simulink model "Test"  (R2022b)
settings: Solver=VariableStepAuto  StartTime=0.0  StopTime=500  MaxStep=0.01  MinStep=1e-3  RelTol=1e-3
settings Model: DataDictionary=Library_Dictionary.sldd  Creator=niklas.baglikow  LastModifiedBy=niklas.baglikow

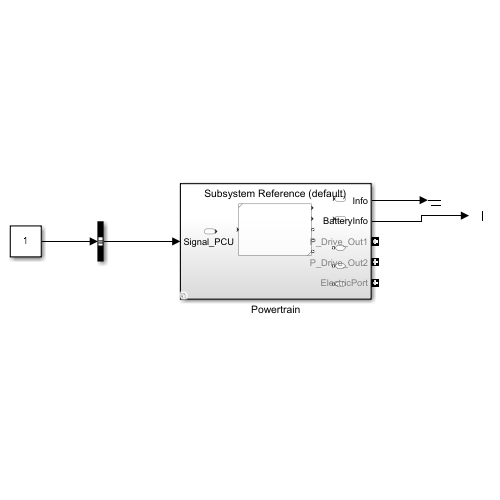
[thumbnail: Simulink's stored preview of the top-level diagram]
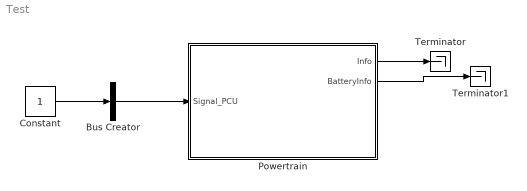
== system Test ==
  Bus Creator : BusCreator  Inputs=1  OutDataTypeStr=Bus: Signal_PCU
  Constant : Constant
  Powertrain : Subsystem  Variant=on
  Terminator : Terminator
  Terminator1 : Terminator
  wires:
  Bus Creator/1 -> Powertrain/1(Signal_PCU)
  Constant/1 -> Bus Creator/1
  Powertrain/1(Info) -> Terminator/1
  Powertrain/2(BatteryInfo) -> Terminator1/1

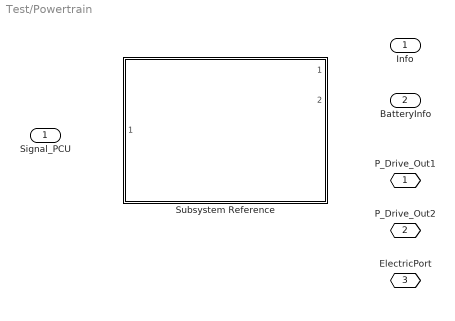
== system Test/Powertrain ==
  Signal_PCU : Inport  OutDataTypeStr=Bus: Signal_PCU
  Subsystem Reference : Subsystem  VariantControl=(default)  ReferencedSubsystem=PowertrainSubsystem
  P_Drive_Out1 : PMIOPort  Side=Right
  P_Drive_Out2 : PMIOPort  Port=2  Side=Right
  ElectricPort : PMIOPort  Port=3  Side=Right
  Info : Outport
  BatteryInfo : Outport  Port=2  OutDataTypeStr=Bus: Signal_Battery
